simulink model "BilinearTranformation"  (R2020b)
settings: Solver=VariableStepAuto  StartTime=0.0  StopTime=10.0  RelTol=1e-3
settings Model: Creator=DELL  LastModifiedBy=DELL

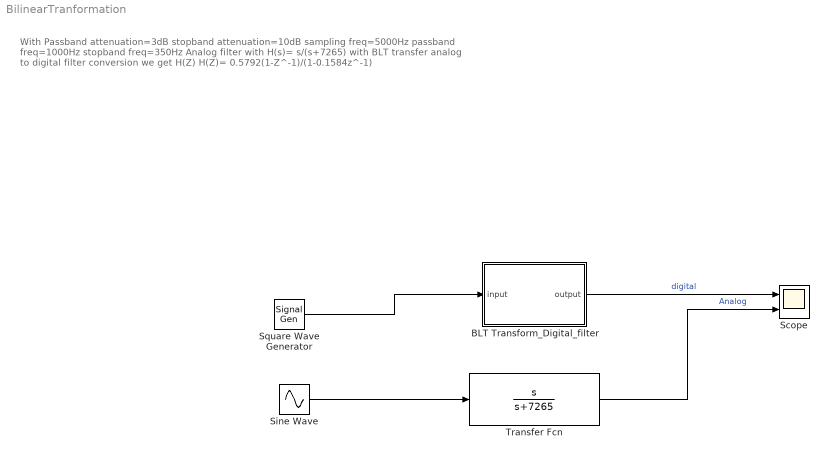
== system BilinearTranformation ==
  note: With Passband attenuation=3dB
      | stopband attenuation=10dB
      | sampling freq=5000Hz
      | passband freq=1000Hz
      | stopband freq=350Hz
      | Analog filter with H(s)= s/(s+7265)
      | with BLT transfer analog to digital filter conversion we get H(Z)
      | H(Z)= 0.5792(1-Z^-1)/(1-0.1584z^-1)
  BLT Transform_Digital_filter : Subsystem
  Scope : Scope  NumInputPorts=2
  Sine Wave : Sin  Frequency=18840  SampleTime=0
  Square Wave Generator : SignalGenerator  WaveForm=square  Frequency=2  Units=rad/sec
  Transfer Fcn : TransferFcn  Numerator=[1 0]  Denominator=[1 7265]
  wires:
  Transfer Fcn/1 -> Scope/2  "Analog"
  Sine Wave/1 -> Transfer Fcn/1
  Square Wave Generator/1 -> BLT Transform_Digital_filter/1(input)
  BLT Transform_Digital_filter/1(output) -> Scope/1  "digital"

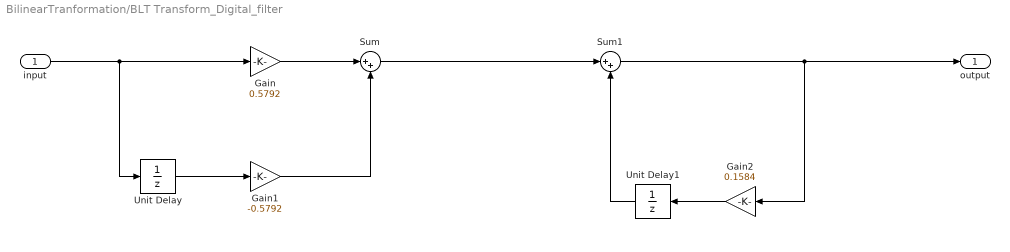
== system BilinearTranformation/BLT Transform_Digital_filter ==
  input : Inport
  Gain : Gain  Gain=0.5792
  Gain1 : Gain  Gain=-0.5792
  Gain2 : Gain  Gain=0.1584
  Sum : Sum  Inputs=|++
  Sum1 : Sum  Inputs=|++
  Unit Delay : UnitDelay  SampleTime=-1  HasFrameUpgradeWarning=on
  Unit Delay1 : UnitDelay  SampleTime=-1  HasFrameUpgradeWarning=on
  output : Outport
  wires:
  Unit Delay/1 -> Gain1/1
  Sum/1 -> Sum1/1
  Gain2/1 -> Unit Delay1/1
  Gain1/1 -> Sum/2
  Gain/1 -> Sum/1
  input/1 -> Unit Delay/1, Gain/1
  Unit Delay1/1 -> Sum1/2
  Sum1/1 -> output/1, Gain2/1
